simulink library "bcm"  (R2021b)
settings: Solver=VariableStepAuto  StartTime=0.0  StopTime=10.0  RelTol=1e-3
undefined symbols (not defined in the file): ENUM_ANTITHEFT_ALARM, ENUM_ANTITHEFT_ARM, ENUM_ANTITHEFT_DISARM, ENUM_ANTITHEFT_WAIT, ENUM_GEARPOSNTOCAN_P, ENUM_PDKEYRAWLULOCK_INUNLOCK, ENUM_PDKEYRAWPS_INPS, ENUM_POWERSTA_ON, ENUM_POWERSTA_READY, ENUM_POWERSTA_STANDBY, ENUM_PWRSTASW_ON, ENUM_PWRSTASW_READY, ENUM_SYSMODE_DEVELOPING, ENUM_SYSMODE_PRODUCT, ENUM_VEHICLETYPE_D21, ENUM_VEHICLETYPE_D31F25, ENUM_VEHICLETYPE_D31HAWD, ENUM_VEHICLETYPE_D31HRWD, ENUM_VEHICLETYPE_D31L24, FALSE, KBCM_ACCSwcPrsTmr_s, KBCM_ALMBrightnessDark_enum, KBCM_AmbBlue_enum, KBCM_AmbBreathT_ms, KBCM_AmbGreen_enum, KBCM_AmbMidPple_enum, KBCM_AmbRed_enum, KBCM_AmbTempCtrlEN_flg, KBCM_AmbTempT_s, KBCM_AmbWelModeENWait_s, KBCM_Antitheft_enum_ovrdflg, KBCM_Antitheft_enum_ovrdval, KBCM_APMDoorCtrlSta_flg_ovrdflg, KBCM_APMDoorCtrlSta_flg_ovrdval, KBCM_CmdKeepT_s, KBCM_CSWLightRstDebT_s, KBCM_CSWTurnLPRstT_s, KBCM_CycleTimeSet_s, KBCM_DelayTSW_flg, KBCM_DiagDRLOFF_flg, KBCM_DiagFLTC_mA, KBCM_DiagFMHT_s, KBCM_DiagFRTC_mA, KBCM_DiagRLTC_mA, KBCM_DiagRRTC_mA, KBCM_DrAPMRetryTimes_cnt, KBCM_DrOpenWdwOT_s, KBCM_DrOpenWdwReady_s, KBCM_DutyCycleSet_cnt, KBCM_DutyOverride_flg, KBCM_DutyOverride_val, KBCM_ESSOffT_ms, KBCM_ESSOnT_ms, KBCM_FDCDKCReDetectT_K, KBCM_FDCDKCUSSFilterT_K, KBCM_HandleLampKeepT_s, KBCM_IVIRstHoldT_ms, KBCM_IVIRstTriggerT_ms, KBCM_ONDelayT_ms, KBCM_RAPSAbnFlashOFFT_ms ... (+51)
libraries: simulink x402, $bdroot x10, hcu_lib x2
(part 1 of 14)
settings Model: Creator=user  LastModifiedBy=zack
settings SolverCC: AlgebraicLoopSolver=TrustRegion
settings DebuggingCC: SFMachineParentedDataDiag=warning

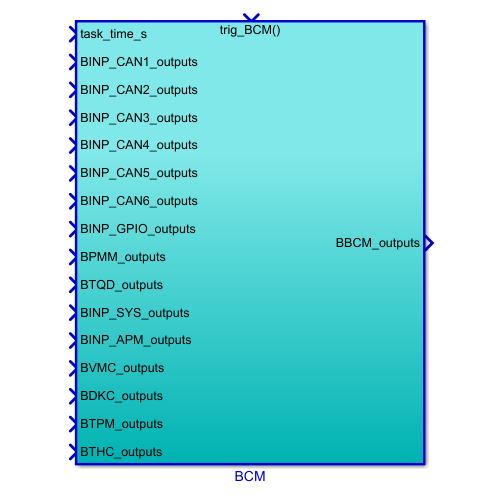
[thumbnail: Simulink's stored preview of the top-level diagram]
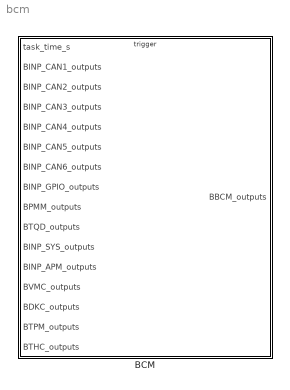
== system bcm ==
  BCM : Subsystem  TreatAsAtomicUnit=on
      settings: RTWSystemCode=Nonreusable function  RTWFcnNameOpts=Use subsystem name  RTWFileNameOpts=Use subsystem name

== system bcm/BCM ==
  task_time_s : Inport
  BINP_CAN1_outputs : Inport  Port=2  OutDataTypeStr=Bus: BINP_CAN1_outputs
  BINP_CAN2_outputs : Inport  Port=3  OutDataTypeStr=Bus: BINP_CAN2_outputs
  BINP_CAN3_outputs : Inport  Port=4  OutDataTypeStr=Bus: BINP_CAN3_outputs
  BINP_CAN4_outputs : Inport  Port=5  OutDataTypeStr=Bus: BINP_CAN4_outputs
  BINP_CAN5_outputs : Inport  Port=6  OutDataTypeStr=Bus: BINP_CAN5_outputs
  BINP_CAN6_outputs : Inport  Port=7  OutDataTypeStr=Bus: BINP_CAN6_outputs
  BINP_GPIO_outputs : Inport  Port=8  OutDataTypeStr=Bus: BINP_GPIO_outputs
  BPMM_outputs : Inport  Port=9  OutDataTypeStr=Bus: BPMM_outputs
  BTQD_outputs : Inport  Port=10  OutDataTypeStr=Bus: BTQD_outputs
  BINP_SYS_outputs : Inport  Port=11  OutDataTypeStr=Bus: BINP_SYS_outputs
  BINP_APM_outputs : Inport  Port=12  OutDataTypeStr=Bus: BINP_APM_outputs
  BVMC_outputs : Inport  Port=13  OutDataTypeStr=Bus: BVMC_outputs
  BDKC_outputs : Inport  Port=14  OutDataTypeStr=Bus: BDKC_outputs
  BTPM_outputs : Inport  Port=15  OutDataTypeStr=Bus: BTPM_outputs
  BTHC_outputs : Inport  Port=16  OutDataTypeStr=Bus: BTHC_outputs
  trig_BCM : TriggerPort  TriggerType=function-call  VariantControl=(inherit)
  BCM : Subsystem
  Bus Creator : BusCreator  Inputs=185  OutDataTypeStr=Bus: BBCM_outputs  NonVirtualBus=on
  Bus Selector : BusSelector  OutputSignals=VINP_HoodSW_flg,VINP_TailgateSW_flg,VINP_DrDoorSW_flg,VINP_PsDoorSW_flg,VINP_RLDoorSW_flg,VINP_RRDoorSW_flg,VINP_TrunkHanSW_flg,VINP_HazardSW_flg,VINP_CentralDoorLockSW_flg,VINP_BrakeSWGPIO_flg,VINP_SeatSW_flg
  Bus Selector1 : BusSelector  OutputSignals=VPMM_PowerSta_enum
  Bus Selector10 : BusSelector  OutputSignals=VTPM_TPMSTLCmd_flg
  Bus Selector11 : BusSelector  OutputSignals=VDKC_KeyAreaLockUnlock_enum,VDKC_KeyAreaPTG_enum,VDKC_KeyAreaPS_enum,VDKC_PCommandToBCM_enum,VDKC_KeyAreaSPTGSta_enum,VDKC_DKeyWelcomeSta_enum
  Bus Selector12 : BusSelector  OutputSignals=VINP_PCommandToBCM_enum,VINP_PDKeyAreaPTG_enum
  Bus Selector13 : BusSelector  OutputSignals=VTHC_Z1TUP_flg,VTHC_Z2TUP_flg,VTHC_Z1TDN_flg,VTHC_Z2TDN_flg
  Bus Selector14 : BusSelector  OutputSignals=VINP_SetUnlockSingle_flg,VINP_IVIStatus_flg,VINP_IVINightModeSta_flg,VINP_HeadLampSW_enum,VINP_RFogLampSW_flg,VINP_FollowMeSW_flg,VINP_IVIRRDefReq_flg,VINP_IVIWIMAINSW_flg,VINP_CANMsgValidIVI2_flg,VINP_CDLUnlockButt_flg,VINP_CDLLockButt_flg,VINP_RoomLampMode_flg,VINP_MFRDNBrightReq_pct,VINP_METERKPHCalcu_kph,VINP_IVIPWModeReq_enum,VINP_AmbLighLowBatAlertSW_flg,VINP_AmbLighSafetyAlertSW_flg,VINP_AmbLightBrightnessSet_enum,VINP_AmbLightDimInDarkSW_flg,VINP_AmbLightSW_flg,VINP_AmbLightWlcmLightSW_flg,VINP_LINKtoDrive_flg,VINP_AmbLightColorSet_enum,VINP_IVIPTGUSStaSW_flg,VINP_LDrvControlCommand_pct,VINP_LPasControlCommand_pct,VINP_LRLDControlCommand_pct,VINP_LRRDControlCommand_pct,VINP_OpenDrOpenWdoSW_flg,VINP_CANMsgValidIVI1_flg,VINP_UserSet_enum,VINP_TurnSwTimeSet_enum,VINP_IVILockSoundSWSta_flg,VINP_ApproachUnlockSW_flg,VINP_WalkawayLockSW_flg,VINP_IVIFrTrunkUnlockReqSta_flg,VINP_IVIPTGOpenHeight_enum,VINP_HMIBCMPostDefogBtnCmd_flg,VINP_IVIStoppingUnlockSWSta_flg,VINP_IVIDrivingLockSWSta_flg,VINP_SenstivityPosition_enum,VINP_IVIHMICustmiKEYSta_enum,VINP_IVIHMICustmiFunSta_enum,VINP_IVIAutoWipHSpdSWCmd_flg,VINP_IVISWCRUndefinedSta_enum,VINP_HMIAutoInterLightCmd_flg,VINP_IVISnowModeCmd_flg,VINP_OFFACMODE_enum,VINP_IVICarWashModeCmd_flg,VINP_IVIMirrorFoldedSWSta_flg,VINP_IVICLWinLockDoorSWSta_flg,VINP_WlcmLightMode_enum
  Bus Selector15 : BusSelector  OutputSignals=VINP_FDCConnDrvWdwCtrlCmd_pct,VINP_FDCConnPasWdwCtrlCmd_pct,VINP_FDCConnRLDWdwCtrlCmd_pct,VINP_FDCConnRRDWdwCtrlCmd_pct
  Bus Selector2 : BusSelector  OutputSignals=VINP_DrLockSta_flg,VINP_CSWDimSw_flg,VINP_CSWPassSWSta_flg,VINP_RLSLampSta_flg,VINP_CSWTurnSwSta_enum,VINP_RLTurnLampC_mA,VINP_RRTurnLampC_mA,VINP_FLTurnLampC_mA,VINP_FRTurnLampC_mA,VINP_MIRRORFOLDSW_flg,VINP_CSWFWasSwSta_enum,VINP_CSWFWipSwSta_enum,VINP_RLSRainSnrWiperCmd_enum,VINP_FWiperAS_flg,VINP_CSWRWipIntSwSta_enum,VINP_RWiperAS_flg,VINP_CSWRWasSWSta_enum,VINP_PTGRDILSta_enum,VINP_RWiperProtection_flg,VINP_FWiperProtection_flg,VINP_SWCmodeSta_flg,VINP_CANMsgValidDKC1_flg,VINP_CANMsgValidZONEDR1_flg,VINP_CANMsgValidZONEFR1_flg,VINP_PTGInnerSW2_enum,VINP_LDrvValWdwOpened_pct,VINP_LPasValWdwOpened_pct,VINP_LRLDValWdwOpened_pct,VINP_LRRDValWdwOpened_pct,VINP_BDDoorFHandleCloseSta_flg,VINP_BPDoorFHandleCloseSta_flg,VINP_BDDoorRHandleCloseSta_flg,VINP_BPDoorRHandleCloseSta_flg,VINP_FLTurnLPErr_flg,VINP_FRTurnLPErr_flg,VINP_RLTurnLPErr_flg,VINP_RRTurnLPErr_flg,VINP_ZFRBCMHRLTurnLPNormalSta_flg,VINP_ZFRBCMHRRTurnLPHNormalSta_flg,VINP_CANMsgValidBodyZonePS1_flg,VINP_BPPTGRDILCmd_enum,VINP_BPPTGIsSetHeightSta_flg,VINP_BPPTGLeftHallPosnSta_enum,VINP_CANMsgValidzGWLINDr1_flg,VINP_SWC2LRightSta_flg,VINP_SWC2LLeftSta_flg,VINP_PTGIsSetHeight_flg,VINP_DKCPDkeyAreaRAPSSta_enum,VINP_CANMsgValidBodyZonePS1_flg,VINP_LeftHallPos_enum,VINP_SWC2RCustomizeSta_flg,VINP_BDAPMWinFOpenedSta_pct,VINP_BDAPMWinROpenedSta_pct,VINP_BPAPMWinFOpenedSta_pct,VINP_BPAPMWinROpenedSta_pct
  Bus Selector3 : BusSelector  OutputSignals=VINP_VehSpeed_kph,VINP_AirBagFailCmd_flg,VINP_ActBrkLampSta_flg,VINP_ESSActive_flg,VINP_SASAngle_Deg
  Bus Selector4 : BusSelector  OutputSignals=VTQD_ShiftGearPosn_enum,VTQD_CrashDetd_flg,VTQD_DiagHCrash_flg,VTQD_ReBrakeLPReq_flg,VTQD_SpdCtrlMode_enum,VTQD_SysMode_enum,VTQD_ComboKeyEn_flg
  Bus Selector5 : BusSelector  OutputSignals=VINP_ReDoorLock_enum,VINP_ReOutsideMirror_enum
  Bus Selector6 : BusSelector  OutputSignals=VINP_FlashAntitheft_enum,VINP_FlashCountAlarm_enum,VINP_FlashMFSWTri_flg,VINP_FlashMirrorFlodPos_flg,VINP_FlashFuelDoorPos_flg,VINP_FlashMFRDNBrightReq_pct,VINP_FlashWiperFixMode_flg,VINP_FlashIVIPTGUSStaSW_enum,VINP_FlashHoodSW_flg,VINP_FlashTailgateSW_flg,VINP_FlashCTDLockSW_flg,VINP_FlashTailgateHDSW_flg,VINP_FlashAPMDoorControlSta_flg,VINP_FlashfUnlockSingle_flg,VINP_FlashAmbFunEN_enum,VINP_FlashAmbWelEN_enum,VINP_FlashAmbDimEN_enum,VINP_FlashAmbLinkDriSta_enum,VINP_FlashAmbPwrWarnEN_enum,VINP_FlashAmbODAEN_enum,VINP_FlashAmbColorSta1_enum,VINP_FlashAmbColorSta2_enum,VINP_FlashAmbColorSta3_enum,VINP_FlashAmbColorSta4_enum,VINP_FlashAmbColorSta5_enum,VINP_FlashAmbColorSta7_enum,VINP_FlashAmbBrightnessSta1_enum,VINP_FlashAmbBrightnessSta2_enum,VINP_FlashAmbBrightnessSta3_enum,VINP_FlashAmbBrightnessSta4_enum,VINP_FlashAmbBrightnessSta5_enum,VINP_FlashAmbBrightnessSta7_enum,VINP_FlashTurnSwTSet123_enum,VINP_FlashTurnSwTSet457_enum,VINP_funAuto_flg,VINP_DiagDRLOFF_flg,VINP_DiagFMHT_s,VINP_DiagFLTC_mA,VINP_DiagFRTC_mA,VINP_DiagRLTC_mA,VINP_DiagRRTC_mA,VINP_FlashWalkOutLkEN_enum,VINP_FlashWalkInUnLkEN_enum,VINP_FlashRoomLampMode_enum,VINP_FlashLockSetting_enum,VINP_FlashFollowMeENFun_enum,VINP_FlashPTGUserHeight1_cnt,VINP_FlashPTGUserHeight2_cnt,VINP_FlashPTGUserHeight3_cnt,VINP_FlashPTGUserHeight4_cnt,VINP_FlashPTGUserHeight5_cnt,VINP_FlashPTGUserHeight7_cnt,VINP_FlashPTGOpenHeight12_enum,VINP_FlashPTGOpenHeight34_enum,VINP_FlashPTGOpenHeight57_enum,VINP_WipRLSCmdHoldEN_flg,VINP_WipRLSCmdCutEN_flg,VINP_WipRLSCmdHoldTime_s,VINP_WipRLSCmdCutTime_s,VINP_FlashACCLevelSta12_enum,VINP_FlashACCLevelSta34_enum,VINP_FlashACCLevelSta57_enum,VINP_FlashAutoLock_enum,VINP_FlashAutoUnlock_enum,VINP_VehicleType_enum,VINP_FlashHMIKey1Func_enum,VINP_FlashHMIKey2Func_enum,VINP_FlashHMIKey3Func_enum,VINP_FlashHMIKey4Func_enum,VINP_FlashHMIKey5Func_enum,VINP_FlashHMIKey6Func_enum,VINP_FlashHMIKey7Func_enum,VINP_FlashHMIKey8Func_enum,VINP_FlashAutoWipHSpdEN_flg,VINP_FlashCLWinLockDrSta_enum
  Bus Selector7 : BusSelector  OutputSignals=VINP_PASDRMR_cm,VINP_PASDRML_cm,VINP_RAPSBCMLockReq_flg,VINP_RAPSErrWarnSta_enum,VINP_RAPSBCMLamp_enum,VINP_APSStaSystem_enum
  Bus Selector8 : BusSelector  OutputSignals=VINP_SRRBSDWarnR_enum,VINP_SRRBSDWarnL_enum,VINP_LeftTurnLightReq_flg,VINP_RightTurnLightReq_flg,VINP_ForceLowBeam_enum,VINP_HazardWarningReq_flg,VINP_ADASACCSta_enum,VINP_TimeGapLevel_enum,VINP_SRRODASoundL_flg,VINP_SRRODASoundR_flg,VINP_SRRODAWarnL_enum,VINP_SRRODAWarnR_enum
  Bus Selector9 : BusSelector  OutputSignals=VINP_HVBattSOCDis_pct,VINP_CSW2DimSwSta_flg,VINP_CSW2PassSWSta_flg,VINP_CSW2FWipSwSta_enum,VINP_CSW2FWasSwSta_enum,VINP_CSW2TurnSwSta_enum,VINP_CSW2RWipWasSwSta_enum,VINP_CANMsgValidShifter2_flg
  Ground{,1..3,11..12} (6 alike) : Ground
  Model Info : simulink/Model-Wide Utilities/Model Info  Frame=on  DisplayStringWithTags=$Id: pmm.mdl 130 2021-02-08 12:40:01Z Shawn $  HorizontalTextAlignment=Center  LeftAlignmentValue=0.5
  Terminator{,1..3} (4 alike) : Terminator
  BBCM_outputs : Outport  OutDataTypeStr=Bus: BBCM_outputs  VectorParamsAs1DForOutWhenUnconnected=off
  wires:
  BPMM_outputs/1 -> Bus Selector1/1
  BINP_CAN4_outputs/1 -> [BINP_CAN4_outputs]
  BINP_CAN1_outputs/1 -> [BINP_CAN1_outputs]
  [BINP_CAN1_outputs] -> Bus Selector3/1
  BINP_GPIO_outputs/1 -> [BINP_GPIO_outputs]
  [BINP_GPIO_outputs] -> Bus Selector/1
  BINP_CAN2_outputs/1 -> [BINP_CAN2_outputs]
  BINP_CAN5_outputs/1 -> Terminator3/1
  [BINP_CAN2_outputs] -> Bus Selector14/1
  BTQD_outputs/1 -> Bus Selector4/1
  Bus Selector3/2 -> BCM/3(VINP_AirBagFailCmd_flg)  "<VINP_AirBagFailCmd_flg>"
  Bus Selector3/1 -> BCM/2(VINP_VehSpeed_kph)  "<VINP_VehSpeed_kph>"
  [BINP_CAN4_outputs] -> Bus Selector2/1
  Bus Selector14/9 -> BCM/27(VINP_CANMsgValidIVI2_flg)  "<VINP_CANMsgValidIVI2_flg>"
  Bus Selector14/2 -> BCM/20(VINP_IVIStatus_flg)  "<VINP_IVIStatus_flg>"
  Bus Selector14/3 -> BCM/21(VINP_IVINightModeSta_flg)  "<VINP_IVINightModeSta_flg>"
  Bus Selector14/4 -> BCM/22(VINP_HeadLampSW_enum)  "<VINP_HeadLampSW_enum>"
  Bus Selector14/5 -> BCM/23(VINP_RFogLampSW_flg)  "<VINP_RFogLampSW_flg>"
  Bus Selector14/6 -> BCM/24(VINP_FollowMeSW_flg)  "<VINP_FollowMeSW_flg>"
  Bus Selector14/1 -> BCM/19(VINP_SetUnlockSingle_flg)  "<VINP_SetUnlockSingle_flg>"
  Bus Selector14/7 -> BCM/25(VINP_IVIRRDefReq_flg)  "<VINP_IVIRRDefReq_flg>"
  Bus Selector14/8 -> BCM/26(VINP_IVIWIMAINSW_flg)  "<VINP_IVIWIMAINSW_flg>"
  Bus Selector14/10 -> BCM/28(VINP_CDLUnlockButt_flg)  "<VINP_CDLUnlockButt_flg>"
  Bus Selector14/11 -> BCM/29(VINP_CDLLockButt_flg)  "<VINP_CDLLockButt_flg>"
  Bus Selector14/12 -> BCM/30(VINP_RoomLampMode_flg)  "<VINP_RoomLampMode_flg>"
  Bus Selector14/13 -> BCM/31(VINP_MFRDNBrightReq_pct)  "<VINP_MFRDNBrightReq_pct>"
  Bus Selector14/14 -> BCM/32(VINP_METERKPHCalcu_kph)  "<VINP_METERKPHCalcu_kph>"
  Bus Selector14/15 -> BCM/33(VINP_IVIPWModeReq_enum)  "<VINP_IVIPWModeReq_enum>"
  task_time_s/1 -> BCM/1(task_time_s)
  BINP_CAN6_outputs/1 -> [BINP_CAN6_outputs]
  [BINP_CAN6_outputs] -> Bus Selector8/1
  Bus Selector8/3 -> BCM/9(VINP_LeftTurnReq_flg)  "<VINP_LeftTurnLightReq_flg>"
  Bus Selector8/4 -> BCM/10(VINP_RightTurnReq_flg)  "<VINP_RightTurnLightReq_flg>"
  Bus Selector8/5 -> BCM/11(VINP_ForceLowBeam_enum)  "<VINP_ForceLowBeam_enum>"
  Bus Selector8/6 -> BCM/12(VINP_HazardWarningReq_flg)  "<VINP_HazardWarningReq_flg>"
  Bus Selector3/3 -> BCM/4(VINP_ActBrkLampSta_flg)  "<VINP_ActBrkLampSta_flg>"
  Bus Selector3/4 -> BCM/5(VINP_ESSActive_flg)  "<VINP_ESSActive_flg>"
  Bus Selector8/1 -> BCM/7(VINP_SRRBSDWarnR_enum)  "<VINP_SRRBSDWarnR_enum>"
  Bus Selector8/2 -> BCM/8(VINP_SRRBSDWarnL_enum)  "<VINP_SRRBSDWarnL_enum>"
  Bus Selector14/24 -> BCM/42(VINP_IVIPTGUSStaSW_flg)  "<VINP_IVIPTGUSStaSW_flg>"
  Bus Selector14/25 -> BCM/43(VINP_LDrvControlCommand_pct)  "<VINP_LDrvControlCommand_pct>"
  Bus Selector14/26 -> BCM/44(VINP_LPasControlCommand_pct)  "<VINP_LPasControlCommand_pct>"
  Bus Selector14/27 -> BCM/45(VINP_LRLDControlCommand_pct)  "<VINP_LRLDControlCommand_pct>"
  Bus Selector14/28 -> BCM/46(VINP_LRRDControlCommand_pct)  "<VINP_LRRDControlCommand_pct>"
  Bus Selector14/29 -> BCM/47(VINP_OpenDrOpenWdoSW_flg)  "<VINP_OpenDrOpenWdoSW_flg>"
  Bus Selector2/1 -> BCM/83(VINP_DrLockSta_flg)  "<VINP_DrLockSta_flg>"
  Bus Selector2/2 -> BCM/84(VINP_CSWDimSw_flg)  "<VINP_CSWDimSw_flg>"
  Bus Selector2/3 -> BCM/85(VINP_CSWPassSWSta_flg)  "<VINP_CSWPassSWSta_flg>"
  Bus Selector2/4 -> BCM/86(VINP_RLSLampSta_flg)  "<VINP_RLSLampSta_flg>"
  Bus Selector2/5 -> BCM/87(VINP_CSWTurnSWSta_enum)  "<VINP_CSWTurnSwSta_enum>"
  Bus Selector2/6 -> BCM/88(VINP_RLTurnLampC_mA)  "<VINP_RLTurnLampC_mA>"
  Bus Selector2/7 -> BCM/89(VINP_RRTurnLampC_mA)  "<VINP_RRTurnLampC_mA>"
  Bus Selector2/8 -> BCM/90(VINP_FLTurnLampC_mA)  "<VINP_FLTurnLampC_mA>"
  Bus Selector2/9 -> BCM/91(VINP_FRTurnLampC_mA)  "<VINP_FRTurnLampC_mA>"
  Bus Selector2/10 -> BCM/92(VINP_MIRRORFOLDSW_flg)  "<VINP_MIRRORFOLDSW_flg>"
  Bus Selector2/11 -> BCM/93(VINP_CSWFWasSWSta_enum)  "<VINP_CSWFWasSwSta_enum>"
  Bus Selector2/12 -> BCM/94(VINP_CSWFWipSWSta_enum)  "<VINP_CSWFWipSwSta_enum>"
  Bus Selector2/13 -> BCM/95(VINP_RLSRainSnrWiperCmd_enum)  "<VINP_RLSRainSnrWiperCmd_enum>"
  Bus Selector2/14 -> BCM/96(VINP_FWiperAS_flg)  "<VINP_FWiperAS_flg>"
  Bus Selector2/15 -> BCM/97(VINP_CSWRWipIntSwSta_enum)  "<VINP_CSWRWipIntSwSta_enum>"
  Bus Selector2/16 -> BCM/98(VINP_RWiperAS_flg)  "<VINP_RWiperAS_flg>"
  Bus Selector2/17 -> BCM/99(VINP_CSWRWasSWSta_enum)  "<VINP_CSWRWasSWSta_enum>"
  Bus Selector2/18 -> BCM/100(VINP_PTGRDILsta_enum)  "<VINP_PTGRDILSta_enum>"
  Bus Selector2/19 -> BCM/101(VINP_RWiperProtection_flg)  "<VINP_RWiperProtection_flg>"
  Bus Selector2/20 -> BCM/102(VINP_FWiperProtection_flg)  "<VINP_FWiperProtection_flg>"
  Bus Selector2/21 -> BCM/103(VINP_SWCmodeSta_flg)  "<VINP_SWCmodeSta_flg>"
  Bus Selector2/22 -> BCM/104(VINP_CANMsgValidDKC1_flg)  "<VINP_CANMsgValidDKC1_flg>"
  Bus Selector2/23 -> BCM/105(VINP_CANMsgValidGWZoneDR1_flg)  "<VINP_CANMsgValidZONEDR1_flg>"
  Bus Selector2/24 -> BCM/106(VINP_CANMsgValidGWZoneFR1_flg)  "<VINP_CANMsgValidZONEFR1_flg>"
  Bus Selector2/25 -> BCM/107(VINP_PTGInnerSW2_enum)  "<VINP_PTGInnerSW2_enum>"
  Bus Selector2/26 -> BCM/108(VINP_LDrvValWdwOpened_pct)  "<VINP_LDrvValWdwOpened_pct>"
  Bus Selector2/27 -> BCM/109(VINP_LPasValWdwOpened_pct)  "<VINP_LPasValWdwOpened_pct>"
  Bus Selector2/28 -> BCM/110(VINP_LRLDValWdwOpened_pct)  "<VINP_LRLDValWdwOpened_pct>"
  Bus Selector2/29 -> BCM/111(VINP_LRRDValWdwOpened_pct)  "<VINP_LRRDValWdwOpened_pct>"
  Bus Selector5/1 -> BCM/148(VINP_ReDoorLock_enum)  "<VINP_ReDoorLock_enum>"
  Bus Selector5/2 -> BCM/149(VINP_ReOutsideMirror_enum)  "<VINP_ReOutsideMirror_enum>"
  Bus Selector/1 -> BCM/150(VINP_HoodSW_flg)  "<VINP_HoodSW_flg>"
  Bus Selector/2 -> BCM/151(VINP_TailgateSW_flg)  "<VINP_TailgateSW_flg>"
  Bus Selector/3 -> BCM/152(VINP_DrDoorSW_flg)  "<VINP_DrDoorSW_flg>"
  Bus Selector/4 -> BCM/153(VINP_PsDoorSW_flg)  "<VINP_PsDoorSW_flg>"
  Bus Selector/5 -> BCM/154(VINP_RLDoorSW_flg)  "<VINP_RLDoorSW_flg>"
  Bus Selector/6 -> BCM/155(VINP_RRDoorSW_flg)  "<VINP_RRDoorSW_flg>"
  Bus Selector/7 -> BCM/156(VINP_TrunkHanSW_flg)  "<VINP_TrunkHanSW_flg>"
  Bus Selector/8 -> BCM/157(VINP_HazardSW_flg)  "<VINP_HazardSW_flg>"
  Bus Selector/9 -> BCM/158(VINP_CentralDoorLockSW_flg)  "<VINP_CentralDoorLockSW_flg>"
  Bus Selector/10 -> BCM/159(VINP_BrakeSWGPIO_flg)  "<VINP_BrakeSWGPIO_flg>"
  Bus Selector1/1 -> BCM/161(VPMM_PwrSta_enum)  "<VPMM_PowerSta_enum>"
  Bus Selector4/1 -> BCM/162(VTQD_ShiftGearPosn_enum)  "<VTQD_ShiftGearPosn_enum>"
  Bus Selector4/2 -> BCM/163(VTQD_CrashDetd_flg)  "<VTQD_CrashDetd_flg>"
  Bus Selector4/3 -> BCM/164(VTQD_DiagHCrash_flg)  "<VTQD_DiagHCrash_flg>"
  Bus Selector4/4 -> BCM/165(VTQD_ReBrakeLPReq_flg)  "<VTQD_ReBrakeLPReq_flg>"
  Bus Selector6/1 -> BCM/169(VINP_FlashAntitheft_enum)  "<VINP_FlashAntitheft_enum>"
  Bus Selector6/2 -> BCM/170(VINP_FlashCountAlarm_enum)  "<VINP_FlashCountAlarm_enum>"
  Bus Selector6/3 -> BCM/171(VINP_FlashMFSWTri_flg)  "<VINP_FlashMFSWTri_flg>"
  Bus Selector6/4 -> BCM/172(VINP_FlashMirrorFlodPos)  "<VINP_FlashMirrorFlodPos_flg>"
  Bus Selector6/5 -> BCM/173(VINP_FlashFuelDoorPos)  "<VINP_FlashFuelDoorPos_flg>"
  Bus Selector6/6 -> BCM/174(VINP_FlashMFRDNBrightReq_pct)  "<VINP_FlashMFRDNBrightReq_pct>"
  Bus Selector6/7 -> BCM/175(VINP_FlashWiperFixMode_flg)  "<VINP_FlashWiperFixMode_flg>"
  Bus Selector6/8 -> BCM/176(VINP_FlashIVIPTGUSStaSW_enum)  "<VINP_FlashIVIPTGUSStaSW_enum>"
  Bus Selector6/9 -> BCM/177(VINP_FlashHoodSW_flg)  "<VINP_FlashHoodSW_flg>"
  Bus Selector6/10 -> BCM/178(VINP_FlashTailgateSW_flg)  "<VINP_FlashTailgateSW_flg>"
  Bus Selector6/11 -> BCM/179(VINP_FlashCTDLockSW_flg)  "<VINP_FlashCTDLockSW_flg>"
  Bus Selector6/12 -> BCM/180(VINP_FlashTailgateHDSW_flg)  "<VINP_FlashTailgateHDSW_flg>"
  Bus Selector6/13 -> BCM/181(VINP_FlashAPMDoorControlSta_flg)  "<VINP_FlashAPMDoorControlSta_flg>"
  Ground11/1 -> BCM/255(VDDM_HVRlyOpCFS_flg)
  Ground12/1 -> BCM/256(VDDM_MCUActCFS_flg)
  Bus Creator/1 -> BBCM_outputs/1
  Bus Selector14/22 -> BCM/40(VINP_LINKtoDRIVE_flg)  "<VINP_LINKtoDrive_flg>"
  Bus Selector14/23 -> BCM/41(VINP_AmbLightColorSet_enum)  "<VINP_AmbLightColorSet_enum>"
  Bus Selector14/21 -> BCM/39(VINP_AmbLightWlcmLightSW_flg)  "<VINP_AmbLightWlcmLightSW_flg>"
  Bus Selector14/20 -> BCM/38(VINP_AmbLightSW_flg)  "<VINP_AmbLightSW_flg>"
  Bus Selector14/19 -> BCM/37(VINP_AmbLightDimInDarkSW_flg)  "<VINP_AmbLightDimInDarkSW_flg>"
  Bus Selector14/18 -> BCM/36(VINP_AmbLightBrightnessSet_enum)  "<VINP_AmbLightBrightnessSet_enum>"
  Bus Selector14/17 -> BCM/35(VINP_AmbLighSafetyAlertSW_flg)  "<VINP_AmbLighSafetyAlertSW_flg>"
  Bus Selector14/16 -> BCM/34(VINP_AmbLighLowBatAlertSW_flg)  "<VINP_AmbLighLowBatAlertSW_flg>"
  BINP_CAN3_outputs/1 -> [BINP_CAN3_outputs]
  [BINP_CAN3_outputs] -> Bus Selector9/1
  Bus Selector9/1 -> BCM/75(VINP_HVBattSOCDis_pct)  "<VINP_HVBattSOCDis_pct>"
  Bus Selector14/30 -> BCM/48(VINP_CANMsgValidIVI1_flg)  "<VINP_CANMsgValidIVI1_flg>"
  Bus Selector6/14 -> BCM/182(VINP_FlashfUnlockSingle_flg)  "<VINP_FlashfUnlockSingle_flg>"
  Bus Selector6/15 -> BCM/183(VINP_FlashAmbFunEN_enum)  "<VINP_FlashAmbFunEN_enum>"
  Bus Selector6/16 -> BCM/184(VINP_FlashAmbWelEN_enum)  "<VINP_FlashAmbWelEN_enum>"
  Bus Selector6/17 -> BCM/185(VINP_FlashAmbDimEN_enum)  "<VINP_FlashAmbDimEN_enum>"
  Bus Selector6/18 -> BCM/186(VINP_FlashAmbLinkDriSta_enum)  "<VINP_FlashAmbLinkDriSta_enum>"
  Bus Selector6/19 -> BCM/187(VINP_FlashAmbPwrWarnEN_enum)  "<VINP_FlashAmbPwrWarnEN_enum>"
  Bus Selector6/20 -> BCM/188(VINP_FlashAmbODAEN_enum)  "<VINP_FlashAmbODAEN_enum>"
  Bus Selector6/21 -> BCM/189(VINP_FlashAmbColorSta1_enum)  "<VINP_FlashAmbColorSta1_enum>"
  Bus Selector6/22 -> BCM/190(VINP_FlashAmbColorSta2_enum)  "<VINP_FlashAmbColorSta2_enum>"
  Bus Selector6/23 -> BCM/191(VINP_FlashAmbColorSta3_enum)  "<VINP_FlashAmbColorSta3_enum>"
  Bus Selector6/24 -> BCM/192(VINP_FlashAmbColorSta4_enum)  "<VINP_FlashAmbColorSta4_enum>"
  Bus Selector6/25 -> BCM/193(VINP_FlashAmbColorSta5_enum)  "<VINP_FlashAmbColorSta5_enum>"
  Bus Selector6/26 -> BCM/194(VINP_FlashAmbColorSta7_enum)  "<VINP_FlashAmbColorSta7_enum>"
  Bus Selector6/27 -> BCM/195(VINP_FlashAmbBrightnessSta1_enum)  "<VINP_FlashAmbBrightnessSta1_enum>"
  Bus Selector6/28 -> BCM/196(VINP_FlashAmbBrightnessSta2_enum)  "<VINP_FlashAmbBrightnessSta2_enum>"
  Bus Selector6/29 -> BCM/197(VINP_FlashAmbBrightnessSta3_enum)  "<VINP_FlashAmbBrightnessSta3_enum>"
  Bus Selector6/30 -> BCM/198(VINP_FlashAmbBrightnessSta4_enum)  "<VINP_FlashAmbBrightnessSta4_enum>"
  Bus Selector6/31 -> BCM/199(VINP_FlashAmbBrightnessSta5_enum)  "<VINP_FlashAmbBrightnessSta5_enum>"
  Bus Selector6/32 -> BCM/200(VINP_FlashAmbBrightnessSta7_enum)  "<VINP_FlashAmbBrightnessSta7_enum>"
  Bus Selector14/31 -> BCM/49(VINP_UserSet_enum)  "<VINP_UserSet_enum>"
  Bus Selector3/5 -> BCM/6(VINP_SASAngle_Deg)  "<VINP_SASAngle_Deg>"
  Bus Selector14/32 -> BCM/50(VINP_TurnSwTimeSet_enum)  "<VINP_TurnSwTimeSet_enum>"
  Bus Selector9/2 -> BCM/76(VINP_CSW2DimSwSta_flg)  "<VINP_CSW2DimSwSta_flg>"
  Bus Selector9/3 -> BCM/77(VINP_CSW2PassSWSta_flg)  "<VINP_CSW2PassSWSta_flg>"
  Bus Selector9/4 -> BCM/78(VINP_CSW2FWipSwSta_enum)  "<VINP_CSW2FWipSwSta_enum>"
  Bus Selector9/5 -> BCM/79(VINP_CSW2FWasSwSta_enum)  "<VINP_CSW2FWasSwSta_enum>"
  Bus Selector9/6 -> BCM/80(VUNP_CSW2TurnSwSta_enum)  "<VINP_CSW2TurnSwSta_enum>"
  Bus Selector9/7 -> BCM/81(VINP_CSW2RWipWasSwSta_enum)  "<VINP_CSW2RWipWasSwSta_enum>"
  Bus Selector14/33 -> BCM/51(VINP_IVILockSoundSWSta_flg)  "<VINP_IVILockSoundSWSta_flg>"
  Bus Selector9/8 -> BCM/82(VINP_CANMsgValidShifter2_flg)  "<VINP_CANMsgValidShifter2_flg>"
  Bus Selector6/33 -> BCM/201(VINP_FlashTurnSwTimeSetSta123_enum)  "<VINP_FlashTurnSwTSet123_enum>"
  Bus Selector6/34 -> BCM/202(VINP_FlashTurnSwTimeSetSta457_enum)  "<VINP_FlashTurnSwTSet457_enum>"
  [BINP_CAN4_outputs] -> Bus Selector12/1
  Bus Selector12/2 -> Terminator1/1  "<VINP_PDKeyAreaPTG_enum>"
  Bus Selector12/1 -> Terminator/1  "<VINP_PCommandToBCM_enum>"
  Bus Selector6/35 -> BCM/203(VINP_funAuto_flg)  "<VINP_funAuto_flg>"
  Bus Selector6/36 -> BCM/204(VINP_DiagDRLOFF_flg)  "<VINP_DiagDRLOFF_flg>"
  Bus Selector6/37 -> BCM/205(VINP_DiagFMHT_s)  "<VINP_DiagFMHT_s>"
  Bus Selector6/38 -> BCM/206(VINP_DiagFLTC_mA)  "<VINP_DiagFLTC_mA>"
  Bus Selector6/39 -> BCM/207(VINP_DiagFRTC_mA)  "<VINP_DiagFRTC_mA>"
  Bus Selector6/40 -> BCM/208(VINP_DiagRLTC_mA)  "<VINP_DiagRLTC_mA>"
  Bus Selector6/41 -> BCM/209(VINP_DiagRRTC_mA)  "<VINP_DiagRRTC_mA>"
  BTHC_outputs/1 -> Bus Selector13/1
  Bus Selector13/2 -> BCM/252(VTHC_Z2UP_flg)  "<VTHC_Z2TUP_flg>"
  Bus Selector13/1 -> BCM/251(VTHC_Z1UP_flg)  "<VTHC_Z1TUP_flg>"
  Bus Selector13/3 -> BCM/253(VTHC_Z1DN_flg)  "<VTHC_Z1TDN_flg>"
  Bus Selector13/4 -> BCM/254(VTHC_Z2DN_flg)  "<VTHC_Z2TDN_flg>"
  Bus Selector2/30 -> BCM/112(VINP_FLHandleClose_flg)  "<VINP_BDDoorFHandleCloseSta_flg>"
  Bus Selector2/33 -> BCM/115(VINP_RRHandleClose_flg)  "<VINP_BPDoorRHandleCloseSta_flg>"
  Bus Selector14/34 -> BCM/52(VINP_ApproachUnlockSW_flg)  "<VINP_ApproachUnlockSW_flg>"
  Bus Selector14/35 -> BCM/53(VINP_WalkawayLockSW_flg)  "<VINP_WalkawayLockSW_flg>"
  Bus Selector6/42 -> BCM/210(VINP_FlashWalkOutLkEN_enum)  "<VINP_FlashWalkOutLkEN_enum>"
  Bus Selector6/43 -> BCM/211(VINP_FlashWalkInUnLkEN_enum)  "<VINP_FlashWalkInUnLkEN_enum>"
  Bus Selector6/44 -> BCM/212(VINP_FlashRmLpModeEN_enum)  "<VINP_FlashRoomLampMode_enum>"
  Bus Selector6/45 -> BCM/213(VINP_FlashLockSettingSta_enum)  "<VINP_FlashLockSetting_enum>"
  Bus Selector6/46 -> BCM/214(VINP_FlashFollowMeENFun_enum)  "<VINP_FlashFollowMeENFun_enum>"
  BVMC_outputs/1 -> Terminator2/1  "BVMC_outputs"
  Bus Selector2/34 -> BCM/116(VINP_FLTurnLPErr_flg)  "<VINP_FLTurnLPErr_flg>"
  Bus Selector2/35 -> BCM/117(VINP_FRTurnLPErr_flg)  "<VINP_FRTurnLPErr_flg>"
  Bus Selector2/36 -> BCM/118(VINP_RLTurnLPErr_flg)  "<VINP_RLTurnLPErr_flg>"
  Bus Selector2/37 -> BCM/119(VINP_RRTurnLPErr_flg)  "<VINP_RRTurnLPErr_flg>"
  Bus Selector2/38 -> BCM/120(VINP_HRLTurnLPNormalSta_flg)  "<VINP_ZFRBCMHRLTurnLPNormalSta_flg>"
  Bus Selector2/39 -> BCM/121(VINP_HRRTurnLPHNormalSta_flg)  "<VINP_ZFRBCMHRRTurnLPHNormalSta_flg>"
  Bus Selector14/36 -> BCM/54(VINP_IVIFrTrunkUnlockReqSta_flg)  "<VINP_IVIFrTrunkUnlockReqSta_flg>"
  BTPM_outputs/1 -> Bus Selector10/1
  Bus Selector10/1 -> BCM/250(VTPM_TPMSTLCmd_flg)  "<VTPM_TPMSTLCmd_flg>"
  BDKC_outputs/1 -> Bus Selector11/1  "BDKC_outputs"
  Bus Selector2/40 -> BCM/122(VINP_CANMsgValidZONER1_flg)  "<VINP_CANMsgValidBodyZonePS1_flg>"
  Bus Selector2/41 -> BCM/123(VINP_ZRPTGRDILCmd_enum)  "<VINP_BPPTGRDILCmd_enum>"
  Bus Selector11/3 -> BCM/140(VDKC_PDKeyAreaPS_enum)  "<VDKC_KeyAreaPS_enum>"
  Bus Selector11/4 -> BCM/141(VDKC_PCommandToBCM_enum)  "<VDKC_PCommandToBCM_enum>"
  Bus Selector14/37 -> BCM/55(VINP_IVIPTGOpenHeight_enum)  "<VINP_IVIPTGOpenHeight_enum>"
  Bus Selector6/47 -> BCM/215(VINP_FlashPTGUserHeight1_cnt)  "<VINP_FlashPTGUserHeight1_cnt>"
  Bus Selector6/48 -> BCM/216(VINP_FlashPTGUserHeight2_cnt)  "<VINP_FlashPTGUserHeight2_cnt>"
  Bus Selector6/49 -> BCM/217(VINP_FlashPTGUserHeight3_cnt)  "<VINP_FlashPTGUserHeight3_cnt>"
  Bus Selector6/50 -> BCM/218(VINP_FlashPTGUserHeight4_cnt)  "<VINP_FlashPTGUserHeight4_cnt>"
  Bus Selector6/51 -> BCM/219(VINP_FlashPTGUserHeight5_cnt)  "<VINP_FlashPTGUserHeight5_cnt>"
  Bus Selector6/52 -> BCM/220(VINP_FlashPTGUserHeight7_cnt)  "<VINP_FlashPTGUserHeight7_cnt>"
  Bus Selector2/42 -> BCM/124(VINP_BPPTGIsSetHeightSta_flg)  "<VINP_BPPTGIsSetHeightSta_flg>"
  Bus Selector2/43 -> BCM/125(VINP_PTGLeftHallPosn_cnt)  "<VINP_BPPTGLeftHallPosnSta_enum>"
  Bus Selector6/53 -> BCM/221(VINP_FlashPTGOpenHeight12_enum)  "<VINP_FlashPTGOpenHeight12_enum>"
  Bus Selector6/54 -> BCM/222(VINP_FlashPTGOpenHeight34_enum)  "<VINP_FlashPTGOpenHeight34_enum>"
  Bus Selector6/55 -> BCM/223(VINP_FlashPTGOpenHeight57_enum)  "<VINP_FlashPTGOpenHeight57_enum>"
  Bus Selector14/38 -> BCM/56(VINP_RRDefSta_flg)  "<VINP_HMIBCMPostDefogBtnCmd_flg>"
  Bus Selector2/31 -> BCM/113(VINP_FRHandleClose_flg)  "<VINP_BPDoorFHandleCloseSta_flg>"
  Bus Selector2/32 -> BCM/114(VINP_RLHandleClose_flg)  "<VINP_BDDoorRHandleCloseSta_flg>"
  Bus Selector11/5 -> BCM/142(VDKC_KeyAreaSPTGSta_enum)  "<VDKC_KeyAreaSPTGSta_enum>"
  Bus Selector11/1 -> BCM/138(VDKC_PDKeyAreaLockUnlock_enum)  "<VDKC_KeyAreaLockUnlock_enum>"
  Bus Selector11/2 -> BCM/139(VDKC_PDKeyAreaPTG_enum)  "<VDKC_KeyAreaPTG_enum>"
  Bus Selector8/7 -> BCM/13(VINP_ADASACCSta_enum)  "<VINP_ADASACCSta_enum>"
  Bus Selector8/8 -> BCM/14(VINP_TimeGapLevel_enum)  "<VINP_TimeGapLevel_enum>"
  Bus Selector14/39 -> BCM/57(VINP_IVIStoppingUnlockSWSta_flg)  "<VINP_IVIStoppingUnlockSWSta_flg>"
  Bus Selector14/40 -> BCM/58(VINP_IVIDrivingLockSWSta_flg)  "<VINP_IVIDrivingLockSWSta_flg>"
  Bus Selector14/41 -> BCM/59(VINP_SenstivityPosition_enum)  "<VINP_SenstivityPosition_enum>"
  Bus Selector2/44 -> BCM/126(VINP_CANMsgValidzGWLINDr1_flg)  "<VINP_CANMsgValidzGWLINDr1_flg>"
  Bus Selector2/45 -> BCM/127(VINP_SWC2LRightSta_flg)  "<VINP_SWC2LRightSta_flg>"
  Bus Selector2/46 -> BCM/128(VINP_SWC2LLeftSta_flg)  "<VINP_SWC2LLeftSta_flg>"
  Bus Selector2/47 -> BCM/129(VINP_PTGIsSetHeight_flg)  "<VINP_PTGIsSetHeight_flg>"
  Bus Selector2/48 -> BCM/130(VDKC_PDKeyAreaRAPSSta_enum)  "<VINP_DKCPDkeyAreaRAPSSta_enum>"
  Bus Selector2/49 -> BCM/131(VINP_CANMsgValidBodyZonePS1_flg)  "<VINP_CANMsgValidBodyZonePS1_flg>"
  BINP_APM_outputs/1 -> Bus Selector7/1  "BINP_APM_outputs"
  Bus Selector7/6 -> BCM/249(VINP_APSStaSystem_enum)  "<VINP_APSStaSystem_enum>"
  Bus Selector7/5 -> BCM/248(VINP_RAPSBCMLamp_enum)  "<VINP_RAPSBCMLamp_enum>"
  Bus Selector7/4 -> BCM/247(VINP_RAPSErrWarn_enum)  "<VINP_RAPSErrWarnSta_enum>"
  Bus Selector7/3 -> BCM/246(VINP_RAPSBCMLockReqCmd_flg)  "<VINP_RAPSBCMLockReq_flg>"
  Bus Selector7/2 -> BCM/245(VAPM_PASDRML_cm)  "<VINP_PASDRML_cm>"
  Bus Selector7/1 -> BCM/244(VAPM_PASDRMR_cm)  "<VINP_PASDRMR_cm>"
  Bus Selector4/5 -> BCM/166(VINP_FDCVMCSpdCtrlModeSta_enum)  "<VTQD_SpdCtrlMode_enum>"
  Bus Selector/11 -> BCM/160(VINP_DrSeatSta_enum)  "<VINP_SeatSW_flg>"
  Bus Selector6/56 -> BCM/224(VINP_DiagWipRLSCmdCutEN_flg)  "<VINP_WipRLSCmdHoldEN_flg>"
  Bus Selector6/57 -> BCM/225(VINP_DiagWipRLSCmdHoldEN_flg)  "<VINP_WipRLSCmdCutEN_flg>"
  Bus Selector6/58 -> BCM/226(VINP_DiagRLSCmdHoldTime_s)  "<VINP_WipRLSCmdHoldTime_s>"
  Bus Selector6/59 -> BCM/227(VINP_DiagRLSCmdCutTime_s)  "<VINP_WipRLSCmdCutTime_s>"
  Bus Selector6/60 -> BCM/228(VINP_FlashACCLevelSta12_enum)  "<VINP_FlashACCLevelSta12_enum>"
  Bus Selector6/61 -> BCM/229(VINP_FlashACCLevelSta34_enum)  "<VINP_FlashACCLevelSta34_enum>"
  Bus Selector6/62 -> BCM/230(VINP_FlashACCLevelSta57_enum)  "<VINP_FlashACCLevelSta57_enum>"
  Bus Selector6/63 -> BCM/231(VINP_FlashAutoLock_enum)  "<VINP_FlashAutoLock_enum>"
  Bus Selector6/64 -> BCM/232(VINP_FlashAutoUnlock_enum)  "<VINP_FlashAutoUnlock_enum>"
  Bus Selector11/6 -> BCM/143(VINP_PDKeyWelcome_enum)  "<VDKC_DKeyWelcomeSta_enum>"
  Bus Selector2/50 -> BCM/132(VINP_LeftHallPos_cnt)  "<VINP_LeftHallPos_enum>"
  Bus Selector6/65 -> BCM/233(VINP_VehicleType_enum)  "<VINP_VehicleType_enum>"
  Bus Selector2/51 -> BCM/133(VINP_SWC2RCustomizeSta_flg)  "<VINP_SWC2RCustomizeSta_flg>"
  Bus Selector14/42 -> BCM/60(VINP_IVIHMICustmiKEYSta_enum)  "<VINP_IVIHMICustmiKEYSta_enum>"
  Bus Selector14/43 -> BCM/61(VINP_IVIHMICustmiFunSta_enum)  "<VINP_IVIHMICustmiFunSta_enum>"
  Bus Selector14/44 -> BCM/62(VINP_IVIAutoWipHSpdSWCmd_flg)  "<VINP_IVIAutoWipHSpdSWCmd_flg>"
  Bus Selector14/45 -> BCM/63(VINP_IVISWCRUndefinedSta_enum)  "<VINP_IVISWCRUndefinedSta_enum>"
  Bus Selector14/46 -> BCM/64(VINP_HMIAutoInterLightCmd_flg)  "<VINP_HMIAutoInterLightCmd_flg>"
  Bus Selector6/66 -> BCM/234(VINP_FlashHMIKey1Func_enum)  "<VINP_FlashHMIKey1Func_enum>"
  Bus Selector6/67 -> BCM/235(VINP_FlashHMIKey2Func_enum)  "<VINP_FlashHMIKey2Func_enum>"
  Bus Selector6/68 -> BCM/236(VINP_FlashHMIKey3Func_enum)  "<VINP_FlashHMIKey3Func_enum>"
  Bus Selector6/69 -> BCM/237(VINP_FlashHMIKey4Func_enum)  "<VINP_FlashHMIKey4Func_enum>"
  Bus Selector6/70 -> BCM/238(VINP_FlashHMIKey5Func_enum)  "<VINP_FlashHMIKey5Func_enum>"
  Bus Selector6/71 -> BCM/239(VINP_FlashHMIKey6Func_enum)  "<VINP_FlashHMIKey6Func_enum>"
  Bus Selector6/72 -> BCM/240(VINP_FlashHMIKey7Func_enum)  "<VINP_FlashHMIKey7Func_enum>"
  Bus Selector6/73 -> BCM/241(VINP_FlashHMIKey8Func_enum)  "<VINP_FlashHMIKey8Func_enum>"
  Bus Selector6/74 -> BCM/242(VINP_FlashAutoWipHSpdEN_flg)  "<VINP_FlashAutoWipHSpdEN_flg>"
  Bus Selector14/47 -> BCM/65(VINP_IVISnowModeCmd_flg)  "<VINP_IVISnowModeCmd_flg>"
  Bus Selector8/9 -> BCM/15(VINP_SRRODASoundL_flg)  "<VINP_SRRODASoundL_flg>"
  Bus Selector8/10 -> BCM/16(VINP_SRRODASoundR_flg)  "<VINP_SRRODASoundR_flg>"
  Bus Selector14/48 -> BCM/66(VINP_OFFACMode_enum)  "<VINP_OFFACMODE_enum>"
  Ground/1 -> BCM/144(VINP_DKCDrvWdwCtrlCmd_pct)
  Ground1/1 -> BCM/145(VINP_DKCPasWdwCtrlCmd_pct)
  Ground2/1 -> BCM/146(VINP_DKCRLDWdwCtrlCmd_pct)
  Ground3/1 -> BCM/147(VINP_DKCRRDWdwCtrlCmd_pct)
  Bus Selector14/49 -> BCM/67(VINP_IVICarWashModeCmd_flg)  "<VINP_IVICarWashModeCmd_flg>"
  Bus Selector14/50 -> BCM/68(VINP_IVIMirrorFoldedSWSta_flg)  "<VINP_IVIMirrorFoldedSWSta_flg>"
  Bus Selector14/51 -> BCM/69(VINP_IVICLWinLockDrSW_flg)  "<VINP_IVICLWinLockDoorSWSta_flg>"
  Bus Selector6/75 -> BCM/243(VINP_FlashCLWinLockDrSta_enum)  "<VINP_FlashCLWinLockDrSta_enum>"
  BINP_SYS_outputs/1 -> [BINP_SYS_output]  "BINP_SYS_output"
  [BINP_SYS_output] -> Bus Selector6/1
  [BINP_SYS_output] -> Bus Selector5/1
  [BINP_SYS_output] -> Bus Selector15/1
  Bus Selector15/2 -> BCM/72(VINP_ConnPasWdwCtrlCmd_pct)  "<VINP_FDCConnPasWdwCtrlCmd_pct>"
  Bus Selector15/3 -> BCM/73(VINP_ConnRLDWdwCtrlCmd_pct)  "<VINP_FDCConnRLDWdwCtrlCmd_pct>"
  Bus Selector15/1 -> BCM/71(VINP_ConnDrvWdwCtrlCmd_pct)  "<VINP_FDCConnDrvWdwCtrlCmd_pct>"
  Bus Selector15/4 -> BCM/74(VINP_ConnRRDWdwCtrlCmd_pct)  "<VINP_FDCConnRRDWdwCtrlCmd_pct>"
  Bus Selector14/52 -> BCM/70(VINP_WlcmLightMode_enum)  "<VINP_WlcmLightMode_enum>"
  BCM/1(VBCM_AntitheftSta_enum) -> Bus Creator/1
  BCM/2(VBCM_TailgateRemote_enum) -> Bus Creator/2
  BCM/3(VBCM_HornCtrl_flg) -> Bus Creator/3
  BCM/4(VBCM_AllDoorSW_flg) -> Bus Creator/4
  BCM/5(VBCM_BCMDoorLockSta_flg) -> Bus Creator/5
  BCM/6(VBCM_AntitheftSeatFlod_flg) -> Bus Creator/6
  BCM/7(VBCM_HoodSW_flg) -> Bus Creator/7
  BCM/8(VBCM_TailgateSW_flg) -> Bus Creator/8
  BCM/9(VBCM_DrDoorSW_flg) -> Bus Creator/9
  BCM/10(VBCM_PsDoorSW_flg) -> Bus Creator/10
  BCM/11(VBCM_RLDoorSW_flg) -> Bus Creator/11
  BCM/12(VBCM_RRDoorSW_flg) -> Bus Creator/12
  BCM/13(VBCM_LockSetting_flg) -> Bus Creator/13
  BCM/14(VBCM_FrChargingDoorCtrl_enum) -> Bus Creator/14
  BCM/15(VBCM_RrChargingDoorCtrl_enum) -> Bus Creator/15
  BCM/16(VBCM_CrashSDetd_flg) -> Bus Creator/16
  BCM/17(VBCM_CTDCtrl_enum) -> Bus Creator/17
  BCM/18(VBCM_DoorLockIND_flg) -> Bus Creator/18
  BCM/19(VBCM_CTDLockSW_flg) -> Bus Creator/19
  BCM/20(VBCM_Dimmer_pct) -> Bus Creator/20
  BCM/21(VBCM_DimmerEN_flg) -> Bus Creator/21
  BCM/22(VBCM_PosLamp_flg) -> Bus Creator/22
  BCM/23(VBCM_LBeam_flg) -> Bus Creator/23
  BCM/24(VBCM_HBeam_flg) -> Bus Creator/24
  BCM/25(VBCM_RrFogLamp_flg) -> Bus Creator/25
  BCM/26(VBCM_BrakeLamp_flg) -> Bus Creator/26
  BCM/27(VBCM_ReverseLamp_flg) -> Bus Creator/27
  BCM/28(VBCM_LDRL_flg) -> Bus Creator/28
  BCM/29(VBCM_RDRL_flg) -> Bus Creator/29
  BCM/30(VBCM_LBSD_flg) -> Bus Creator/30
  BCM/31(VBCM_RBSD_flg) -> Bus Creator/31
  BCM/32(VBCM_HazardSW_flg) -> Bus Creator/32
  BCM/33(VBCM_LTurnLP_flg) -> Bus Creator/33
  BCM/34(VBCM_RTurnLP_flg) -> Bus Creator/34
  BCM/35(VBCM_BCMBuzzerReq_flg) -> Bus Creator/35
  BCM/36(VBCM_MirrorCtrl_enum) -> Bus Creator/36
  BCM/37(VBCM_MirrorDefog_flg) -> Bus Creator/37
  BCM/38(VBCM_RrDefog_flg) -> Bus Creator/38
  BCM/39(VBCM_RoomLampH_flg) -> Bus Creator/39
  BCM/40(VBCM_RoomLampL_flg) -> Bus Creator/40
  BCM/41(VBCM_TrunkRel_flg) -> Bus Creator/41
  BCM/42(VBCM_TailgateHDSW_flg) -> Bus Creator/42
  BCM/43(VBCM_FWiperL_flg) -> Bus Creator/43
  BCM/44(VBCM_FWiperH_flg) -> Bus Creator/44
  BCM/45(VBCM_RWiper_flg) -> Bus Creator/45
  BCM/46(VBCM_WasherCtrl_enum) -> Bus Creator/46
  BCM/47(VBCM_WiperFixMode_flg) -> Bus Creator/47
  BCM/48(VBCM_SleepReq_flg) -> Bus Creator/48
  BCM/49(VBCM_AmbLightBreath1_enum) -> Bus Creator/49
  BCM/50(VBCM_AmbLightBreath2_enum) -> Bus Creator/50
  BCM/51(VBCM_AmbLightBreath3_enum) -> Bus Creator/51
  BCM/52(VBCM_AmbLightBreath4_enum) -> Bus Creator/52
  BCM/53(VBCM_AmbLightBreath5_enum) -> Bus Creator/53
  BCM/54(VBCM_AmbLightBreath6_enum) -> Bus Creator/54
  BCM/55(VBCM_AmbLightBrightness1_enum) -> Bus Creator/55
  BCM/56(VBCM_AmbLightBrightness2_enum) -> Bus Creator/56
  BCM/57(VBCM_AmbLightBrightness3_enum) -> Bus Creator/57
  BCM/58(VBCM_AmbLightBrightness4_enum) -> Bus Creator/58
  BCM/59(VBCM_AmbLightBrightness5_enum) -> Bus Creator/59
  BCM/60(VBCM_AmbLightBrightness6_enum) -> Bus Creator/60
  BCM/61(VBCM_AmbLightColor1_enum) -> Bus Creator/61
  BCM/62(VBCM_AmbLightColor2_enum) -> Bus Creator/62
  BCM/63(VBCM_AmbLightColor3_enum) -> Bus Creator/63
  BCM/64(VBCM_AmbLightColor4_enum) -> Bus Creator/64
  BCM/65(VBCM_AmbLightColor5_enum) -> Bus Creator/65
  BCM/66(VBCM_AmbLightColor6_enum) -> Bus Creator/66
  BCM/67(VBCM_LampPwr_flg) -> Bus Creator/67
  BCM/68(VBCM_SPTGDet_flg) -> Bus Creator/68
  BCM/69(VBCM_APSOpenPTG_flg) -> Bus Creator/69
  BCM/70(VBCM_FollowMe_flg) -> Bus Creator/70
  BCM/71(VBCM_IVIRST_flg) -> Bus Creator/71
  BCM/72(VBCM_CountAlarm_enum) -> Bus Creator/72
  BCM/73(VBCM_MFSWTri_flg) -> Bus Creator/73
  BCM/74(VBCM_MirrorFlodPos_flg) -> Bus Creator/74
  BCM/75(VBCM_FuelDoorPos_flg) -> Bus Creator/75
  BCM/76(VBCM_MFRDNBrightReq_pct) -> Bus Creator/76
  BCM/77(VBCM_PTGInnerSW2_enum) -> Bus Creator/77
  BCM/78(VBCM_DiagHCrash_flg) -> Bus Creator/78
  BCM/79(VBCM_DiagFLTS_flg) -> Bus Creator/79
  BCM/80(VBCM_DiagFRTS_flg) -> Bus Creator/80
  BCM/81(VBCM_DiagRLTS_flg) -> Bus Creator/81
  BCM/82(VBCM_DiagRRTS_flg) -> Bus Creator/82
  BCM/83(VBCM_DrvWdwCtrlCmd_pct) -> Bus Creator/83
  BCM/84(VBCM_PasWdwCtrlCmd_pct) -> Bus Creator/84
  BCM/85(VBCM_DrRWdwCtrlCmd_pct) -> Bus Creator/85
  BCM/86(VBCM_PsRWdwCtrlCmd_pct) -> Bus Creator/86
  BCM/87(VBCM_APMDoorControlSta_flg) -> Bus Creator/87
  BCM/88(VBCM_AmbFunEN_flg) -> Bus Creator/88
  BCM/89(VBCM_AmbWelEN_flg) -> Bus Creator/89
  BCM/90(VBCM_AmbDimEN_flg) -> Bus Creator/90
  BCM/91(VBCM_AmbLinkDriSta_flg) -> Bus Creator/91
  BCM/92(VBCM_AmbPwrWarnEN_flg) -> Bus Creator/92
  BCM/93(VBCM_AmbODAEN_flg) -> Bus Creator/93
  BCM/94(VBCM_AmbColorSta_enum) -> Bus Creator/94
  BCM/95(VBCM_AmbBrightSta_enum) -> Bus Creator/95
  BCM/96(VBCM_LockAlarm_enum) -> Bus Creator/96
  BCM/97(VBCM_ATCtrl_enum) -> Bus Creator/97
  BCM/98(VBCM_fUnlockSingle_flg) -> Bus Creator/98
  BCM/99(VBCM_UserNow_enum) -> Bus Creator/99
  BCM/100(VBCM_AmbFunENFlash_enum) -> Bus Creator/100
  BCM/101(VBCM_AmbWelENFlash_enum) -> Bus Creator/101
  BCM/102(VBCM_AmbDimENFlash_enum) -> Bus Creator/102
  BCM/103(VBCM_AmbLinkDriStaFlash_enum) -> Bus Creator/103
  BCM/104(VBCM_AmbPwrWarnENFlash_enum) -> Bus Creator/104
  BCM/105(VBCM_AmbODAENFlash_enum) -> Bus Creator/105
  BCM/106(VBCM_AmbColorSta1_enum) -> Bus Creator/106
  BCM/107(VBCM_AmbColorSta2_enum) -> Bus Creator/107
  BCM/108(VBCM_AmbColorSta3_enum) -> Bus Creator/108
  BCM/109(VBCM_AmbColorSta4_enum) -> Bus Creator/109
  BCM/110(VBCM_AmbColorSta5_enum) -> Bus Creator/110
  BCM/111(VBCM_AmbColorSta7_enum) -> Bus Creator/111
  BCM/112(VBCM_AmbBrightnessSta1_enum) -> Bus Creator/112
  BCM/113(VBCM_AmbBrightnessSta2_enum) -> Bus Creator/113
  BCM/114(VBCM_AmbBrightnessSta3_enum) -> Bus Creator/114
  BCM/115(VBCM_AmbBrightnessSta4_enum) -> Bus Creator/115
  BCM/116(VBCM_AmbBrightnessSta5_enum) -> Bus Creator/116
  BCM/117(VBCM_AmbBrightnessSta7_enum) -> Bus Creator/117
  BCM/118(VBCM_HazardIND_flg) -> Bus Creator/118
  BCM/119(VBCM_DimSwSta_flg) -> Bus Creator/119
  BCM/120(VBCM_PassSWSta_flg) -> Bus Creator/120
  BCM/121(VBCM_FWipSwSta_enum) -> Bus Creator/121
  BCM/122(VBCM_FWasSwSta_enum) -> Bus Creator/122
  BCM/123(VBCM_TurnSwSta_enum) -> Bus Creator/123
  BCM/124(VBCM_TurnSwTSetSta_enum) -> Bus Creator/124
  BCM/125(VBCM_SPTGENFun_flg) -> Bus Creator/125
  BCM/126(VBCM_SPTGENFunMem_enum) -> Bus Creator/126
  BCM/127(VBCM_OutMode_enum) -> Bus Creator/127
  BCM/128(VBCM_TurnSwTimeSetSta123_enum) -> Bus Creator/128
  BCM/129(VBCM_TurnSwTimeSetSta457_enum) -> Bus Creator/129
  BCM/130(VBCM_FDLHandleLampCmd_flg) -> Bus Creator/130
  BCM/131(VBCM_FDRHandleLampCmd_flg) -> Bus Creator/131
  BCM/132(VBCM_FDHandleCmd_enum) -> Bus Creator/132
  BCM/134(VBCM_WalkInUnLkENMem_enum) -> Bus Creator/134
  BCM/135(VBCM_WalkOutLkENMem_enum) -> Bus Creator/135
  BCM/136(VBCM_RmLpModeENMem_enum) -> Bus Creator/136
  BCM/137(VBCM_LockSettingStaMem_enum) -> Bus Creator/137
  BCM/138(VBCM_FollowMeENMem_enum) -> Bus Creator/138
  BCM/139(VBCM_WalkInUnLkEnFunSta_flg) -> Bus Creator/139
  BCM/140(VBCM_WalkOutLkEnFunSta_flg) -> Bus Creator/140
  BCM/141(VBCM_RmLpModeENFunSta_flg) -> Bus Creator/141
  BCM/142(VBCM_FollowMeENFunSta_flg) -> Bus Creator/142
  BCM/143(VBCM_HoodRelCmd_flg) -> Bus Creator/143
  BCM/144(VBCM_WelcomeLight_enum) -> Bus Creator/144
  BCM/145(VBCM_PTGOpenHeightSta_enum) -> Bus Creator/145
  BCM/146(VBCM_UserHeightSet_cnt) -> Bus Creator/146
  BCM/147(VBCM_PTGUserHeight1_cnt) -> Bus Creator/147
  BCM/148(VBCM_PTGUserHeight2_cnt) -> Bus Creator/148
  BCM/149(VBCM_PTGUserHeight3_cnt) -> Bus Creator/149
  BCM/150(VBCM_PTGUserHeight4_cnt) -> Bus Creator/150
  BCM/151(VBCM_PTGUserHeight5_cnt) -> Bus Creator/151
  BCM/152(VBCM_PTGUserHeight7_cnt) -> Bus Creator/152
  BCM/153(VBCM_PTGOpenHeight12_enum) -> Bus Creator/153
  BCM/154(VBCM_PTGOpenHeight34_enum) -> Bus Creator/154
  BCM/155(VBCM_PTGOpenHeight57_enum) -> Bus Creator/155
  BCM/156(VBCM_SenstivityPosnCmd_enum) -> Bus Creator/156
  BCM/157(VBCM_TimeGapLevelSta_enum) -> Bus Creator/157
  BCM/158(VBCM_ACCLevelMem12_enum) -> Bus Creator/158
  BCM/159(VBCM_ACCLevelMem34_enum) -> Bus Creator/159
  BCM/160(VBCM_ACCLevelMem57_enum) -> Bus Creator/160
  BCM/161(VBCM_LRightStaCmd_flg) -> Bus Creator/161
  BCM/162(VBCM_LLeftStaCmd_flg) -> Bus Creator/162
  BCM/163(VBCM_AutoLockSta_flg) -> Bus Creator/163
  BCM/164(VBCM_AutoLockMem_enum) -> Bus Creator/164
  BCM/165(VBCM_AutoUnlockSta_flg) -> Bus Creator/165
  BCM/166(VBCM_AutoUnlockMem_enum) -> Bus Creator/166
  BCM/167(VBCM_HMIKey1FuncSta_enum) -> Bus Creator/167
  BCM/168(VBCM_HMIKey2FuncSta_enum) -> Bus Creator/168
  BCM/169(VBCM_HMIKey3FuncSta_enum) -> Bus Creator/169
  BCM/170(VBCM_HMIKey4FuncSta_enum) -> Bus Creator/170
  BCM/171(VBCM_HMIKey5FuncSta_enum) -> Bus Creator/171
  BCM/172(VBCM_HMIKey6FuncSta_enum) -> Bus Creator/172
  BCM/173(VBCM_HMIKey7FuncSta_enum) -> Bus Creator/173
  BCM/174(VBCM_HMIKey8FuncSta_enum) -> Bus Creator/174
  BCM/175(VBCM_AutoWipHSpdENSta_flg) -> Bus Creator/175
  BCM/176(VBCM_DrvWdwReqAP_enum) -> Bus Creator/176
  BCM/177(VBCM_PasWdwReqAP_enum) -> Bus Creator/177
  BCM/178(VBCM_DrRWdwReqAP_enum) -> Bus Creator/178
  BCM/179(VBCM_PsRWdwReqAP_enum) -> Bus Creator/179
  BCM/180(VBCM_CLWinLockDrSta_flg) -> Bus Creator/180
  BCM/181(VBCM_CLWinLockDrStaMem_enum) -> Bus Creator/181
  BCM/182(VBCM_WinLFOpenedSta_pct) -> Bus Creator/182
  BCM/183(VBCM_WinRFOpenedSta_pct) -> Bus Creator/183
  BCM/184(VBCM_WinLROpenedSta_pct) -> Bus Creator/184
  BCM/185(VBCM_WinRROpenedSta_pct) -> Bus Creator/185
  Bus Selector2/52 -> BCM/134(VINP_BDAPMWinFOpenedSta_pct)  "<VINP_BDAPMWinFOpenedSta_pct>"
  Bus Selector2/53 -> BCM/135(VINP_BDAPMWinROpenedSta_pct)  "<VINP_BDAPMWinROpenedSta_pct>"
  Bus Selector2/54 -> BCM/136(VINP_BPAPMWinFOpenedSta_pct)  "<VINP_BPAPMWinFOpenedSta_pct>"
  Bus Selector2/55 -> BCM/137(VINP_BPAPMWinROpenedSta_pct)  "<VINP_BPAPMWinROpenedSta_pct>"
  Bus Selector8/11 -> BCM/17(VINP_SRRODAWarnL_enum)  "<VINP_SRRODAWarnL_enum>"
  Bus Selector8/12 -> BCM/18(VINP_SRRODAWarnR_enum)  "<VINP_SRRODAWarnR_enum>"
  BCM/133(VBCM_HBeamADB_enum) -> Bus Creator/133
  Bus Selector4/7 -> BCM/168(VTQD_ComboKeyEn_flg)  "<VTQD_ComboKeyEn_flg>"
  Bus Selector4/6 -> BCM/167(VTQD_SysMode_enum)  "<VTQD_SysMode_enum>"
